simulink model "PWMdinamico"  (R2023b)
settings: Solver=VariableStepAuto  StartTime=0.0  StopTime=0.06  RelTol=1e-3
libraries: simulink x1
settings Model: Creator=luisf  LastModifiedBy=luisf

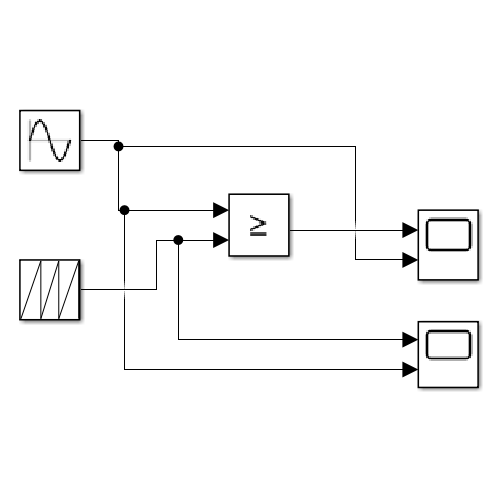
[thumbnail: Simulink's stored preview of the top-level diagram]
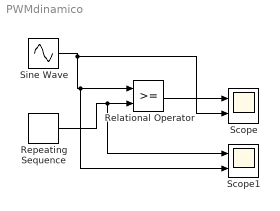
== system PWMdinamico ==
  Relational Operator : RelationalOperator  OutDataTypeStr=boolean  RndMeth=Simplest  InputSameDT=off
  Repeating Sequence : simulink/Sources/Repeating Sequence  rep_seq_t=[0 1/1000]  rep_seq_y=[0 1]
  Scope : Scope  NumInputPorts=2
  Scope1 : Scope  NumInputPorts=2
  Sine Wave : Sin  Amplitude=0.5  Bias=0.5  Frequency=2*pi*50  SampleTime=0
  wires:
  Repeating Sequence/1 -> Scope1/1, Relational Operator/2
  Sine Wave/1 -> Scope/2, Scope1/2, Relational Operator/1
  Relational Operator/1 -> Scope/1
